simulink model "phase_port_simulink"  (R2025a)
settings: Solver=ode15s  StartTime=0.0  StopTime=1.5  RelTol=1e-3
settings Model: Creator=Глеб  LastModifiedBy=Глеб

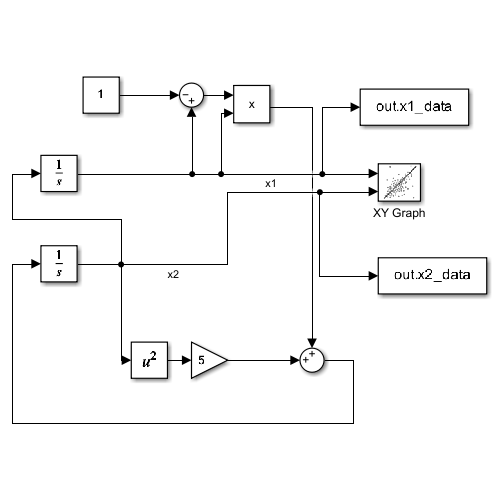
[thumbnail: Simulink's stored preview of the top-level diagram]
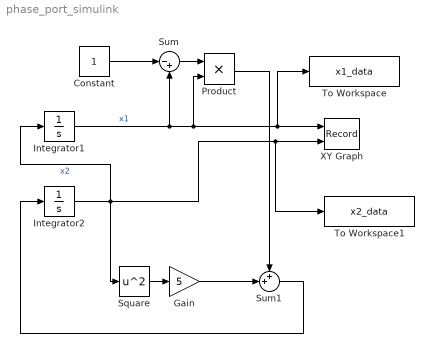
== system phase_port_simulink ==
  Constant : Constant
  Gain : Gain  Gain=5
  Integrator1 : Integrator  InitialCondition=0.1
  Integrator2 : Integrator
  Product : Product
  Square : Math  Operator=square
  Sum : Sum  Inputs=|-+
  Sum1 : Sum  Inputs=++|
  To Workspace : ToWorkspace  VariableName=x1_data  SampleTime=-1
  To Workspace1 : ToWorkspace  VariableName=x2_data  SampleTime=-1
  XY Graph : Record  NumPorts=2.0  FileSettingsInternal="{\"entries\":[{\"content\":{\"excelSettings\":{\"content\":{},\"type\":\"Streamout.ExcelSettings\"},\"parquetSettings\":{\"content\":{},\"type\":\"Streamout.ParquetSettings\"}},\"type\":\"Streamout.FileSettingStorage\",\"uuid\":\"\"}],\"packageUris\":[\"http:\\/\\/schema.mathworks.com\\/mf0\\/streamout_blocks\\/R2020a\"],\"version\":\"1.0\"}"  FrameSettings=[0, 0]  Layout=[1 1]  SignalsInternal="{\"entries\":[{\"content\":{\"signals\":[{\"content\":{\"blockPath\":[],\"dimensions\":[1],\"domain\":\"\",\"lineColor\":\"#0072bd\",\"lineWidth\":2,\"port\":1,\"sid\":[\"\"],\"signalID\":1,\"signalName\":\"x1\"},\"type\":\"RecordBlkView.Signal\",\"uuid\":\"\"},{\"content\":{\"blockPath\":[],\"dimensions\":[1],\"domain\":\"\",\"lineColor\":\"#d95319\",\"lineWidth\":2,\"port\":2,\"sid\":[\"\"],\"signalID\":2,\"signalName\":\"x2\"},\"type\":\"RecordBlkView.Signal\",\"uuid\":\"\"}]},\"type\":\"RecordBlkView.InputSignals\",\"uuid\":\"\"}],\"packageUris\":[\"http:\\/\\/schema.mathworks.com\\/mf0\\/streamout_blocks\\/R2020a\"],\"version\":\"1.0\"}"  VisualizationBindings="{\"xyplotplugin\":{\"info\":[{\"series\":[{\"bindingParametersList\":[{\"parameter\":\"X-Axis\",\"signalID\":574,\"signalName\":\"x1\"},{\"parameter\":\"Y-Axis\",\"signalID\":578,\"signalName\":\"x2\"},{\"parameter\":\"X-Axis\",\"signalID\":574,\"signalName\":\"x1\"},{\"parameter\":\"Y-Axis\",\"signalID\":578,\"signalName\":\"x2\"}],\"seriesID\":0}],\"subplotID\":1}]}}"  CompatibilityTag=XY
  wires:
  Integrator1/1 -> Sum/2, Product/2, To Workspace/1, XY Graph/1  "x1"
  Integrator2/1 -> Integrator1/1, To Workspace1/1, XY Graph/2, Square/1  "x2"
  Square/1 -> Gain/1
  Constant/1 -> Sum/1
  Sum/1 -> Product/1
  Product/1 -> Sum1/1
  Gain/1 -> Sum1/2
  Sum1/1 -> Integrator2/1
